simulink model "IDMF_datagenerator"  (R2022a)
settings: Solver=VariableStepAuto  StartTime=0.0  StopTime=30  FixedStep=0.05  RelTol=1e-3
PostLoadFcn:
  | %Add subfolders to path
  | addpath('virtualworld');
InitFcn:
  | startScript;
values from neighbouring files (symbols this model uses):
  angularVelocity = [0 0 -0.01]    [startScript.m]
  angularVelocityforLanding = [0 0 0]    [startScript.m]
  dronestartlocation = [-1.5 0 4]    [startScript.m]
  Dstar = -0.5    [startScript.m]
  finalHoverHeight = 2.5    [startScript.m]
  helipadLocation = [14 0.6 5]    [startScript.m]
  linearVelocity = [5 0.05 1]    [startScript.m]
  linearVelocityforHover = [0.65 0.05 0.3]    [startScript.m]
  windAVelocity = [0 0.1 0.1]    [startScript.m]
  windLVelocity = [0.1 0 0.3]    [startScript.m]
undefined symbols (not defined in the file or in its folder): fspecial, gcbh, Kanade, Lucas, Rec, SDTV, vrmfunc
libraries: visiontextngfix x11, visionconversions x9, visionanalysis x8, vrlib x7, slpidlib x3, sharedtransform x2, simulink x1
(part 3 of 3)

== matlab function IDMF_datagenerator/ Optical Flow Algorithm for Obstacle Avoidance/Subsystem/MATLAB Function4 ==
  data: points input; vel_Lines output single size=[5000 4]; vel_points output single size=[5000 2]
function [vel_Lines, vel_points]=OpticalFlowLines(points)
%persistent vel_Lines;
rop=round(points*100)/100;
orderedpoints = sortrows(rop);
orderedpoints1 = sortrows(rop,2);
X = [];
Y = [];
shiftX = [];
shiftY=[];
length(orderedpoints)
%(orderedpoints(i,1)==orderedpoints(i+1,1)|| orderedpoints(i,1)==orderedpoints(i+1,1)+1 || orderedpoints(i,1)==orderedpoints(i+1,1)-1 ...
                %|| orderedpoints(i,1)==orderedpoints(i+1,1)+2 || orderedpoints(i,1)==orderedpoints(i+1,1)-2) &&
%|| orderedpoints(i,1)==orderedpoints(i+1,1)+1 || orderedpoints(i,1)==orderedpoints(i+1,1)-1)
if length(orderedpoints)>2
for i = 1:2:length(orderedpoints)-1
    if i ==1 && orderedpoints(i,1)==orderedpoints(i+1,1)
        X = [X ;orderedpoints(i,1)];
        Y = [Y ;orderedpoints(i,2)];
        shiftX = [shiftX ;orderedpoints(i+1,1)];
        shiftY = [shiftY ;orderedpoints(i+1,2)];
    else
        if i ~=1 && (abs(orderedpoints(i,1)-orderedpoints(i+1,1))<3)
        X = [X ;orderedpoints(i,1)];
        Y = [Y ;orderedpoints(i,2)];
        shiftX = [shiftX ;orderedpoints(i+1,1)];
        shiftY = [shiftY ;orderedpoints(i+1,2)];
        
        elseif i~=1 &&  (abs(orderedpoints(i,1)-orderedpoints(i-1,1))<2)
        X = [X ;orderedpoints(i,1)];
        Y = [Y ;orderedpoints(i,2)];
        shiftX = [shiftX ;orderedpoints(i-1,1)];
        shiftY = [shiftY ;orderedpoints(i-1,2)];
    end
    end
end
for i = 1:2:length(orderedpoints1)-1
    if i ==1 && orderedpoints1(i,2)==orderedpoints1(i+1,2)
        X = [X ;orderedpoints1(i,1)];
        Y = [Y ;orderedpoints1(i,2)];
        shiftX = [shiftX ;orderedpoints1(i+1,1)];
        shiftY = [shiftY ;orderedpoints1(i+1,2)];
    else
        if i ~=1 && (abs(orderedpoints1(i,2)-orderedpoints1(i+1,2))<3)
        X = [X ;orderedpoints1(i,1)];
        Y = [Y ;orderedpoints1(i,2)];
        shiftX = [shiftX ;orderedpoints1(i+1,1)];
        shiftY = [shiftY ;orderedpoints1(i+1,2)];
        
        elseif i~=1 &&  (abs(orderedpoints1(i,2)-orderedpoints1(i-1,2))<2)
        X = [X ;orderedpoints1(i,1)];
        Y = [Y ;orderedpoints1(i,2)];
        shiftX = [shiftX ;orderedpoints1(i-1,1)];
        shiftY = [shiftY ;orderedpoints1(i-1,2)];
    end
    end
end
% for i = 1:length(orderedpoints)-1
%     for j=i+1:length(orderedpoints)
%         X = [X ;orderedpoints(i,1)];
%         Y = [Y ;orderedpoints(i,2)];
%         shiftX = [shiftX ;orderedpoints(j,1)];
%         shiftY = [shiftY ;orderedpoints(j,2)];
%     end
% end

    vel_points = [X(:), Y(:); shiftX(:),  shiftY(:) ];
    x= single([X(:), Y(:), shiftX(:),  shiftY(:)]);

else
    vel_points = [points; points];
    x= single([points, points]);
end
vel_Lines=x;
% vel_Lines=padarray(x,50-length(x),0,'post');

== matlab function IDMF_datagenerator/ Optical Flow Algorithm for Obstacle Avoidance/Subsystem/sumele ==
  data: u input; y1 output; n1 output; y2 output; n2 output
function [y1,n1,y2,n2] = fcn(u)
u1=rmoutliers(u);
u2=rmoutliers(u,'percentiles',[30 70]);
n1=length(u1);
n2=length(u2);
% if n1==1
%     y1=0.00;
% else
y1 = double(sum(u1));
% end
y2 = double(sum(u2));
if n2==1
    y2=0.00;
else
y2 = double(sum(u2))/n2;
end

== matlab function IDMF_datagenerator/ Optical Flow Algorithm for Obstacle Avoidance/Subsystem/length1 ==
  data: lines input; l1 output size=5000; l2 output size=5000; N output; reset input; oldlines output size=[5000 4]
function [l1,l2,N,oldlines] = fcn(lines, reset)
l1=single([]);
l2=single([]);
persistent x;
% size(x)
if isempty(x)
    x=lines;
end
if reset>0
    oldlines=x;
else
    oldlines=lines;
end
N = 0;
% size(lines)
if isempty(nonzeros(oldlines))
    oldlines=lines;
end

a1=size(lines);
a1=a1(1,1);
a2=size(oldlines);
a2=a2(1,1);
lines = sortrows(lines);
oldlines=sortrows(oldlines);
% a1=length(lines);
% a2=length(oldlines);
if a1<=a2
for i = 1: a1
    for j = 1:a2
        if abs(lines(i,1) + lines(i,3) - oldlines(j,3) -oldlines(j,1))<=5 && N~=i
           if norm(lines(i,1:2)-lines(i,3:4))~=0 && norm(oldlines(j,1:2)-oldlines(j,3:4))~=0
            l1 = [l1 ;norm(lines(i,1:2)-lines(i,3:4))];
            l2 = [l2; norm(oldlines(j,1:2)-oldlines(j,3:4))];
            N = N+1;
           end
        end
    end
end
else
for i = 1: a2
    for j = 1:a1
        if abs(oldlines(i,1) + oldlines(i,3) - lines(j,3) -lines(j,1))<=5  && N~=i
           if norm(lines(j,1:2)-lines(j,3:4))~=0 && norm(oldlines(i,1:2)-oldlines(i,3:4))~=0
            l1 = [l1 ;norm(lines(j,1:2)-lines(j,3:4))];
            l2 = [l2; norm(oldlines(i,1:2)-oldlines(i,3:4))];
            N = N+1;
           end
        end
    end
end
end
x=lines;

== matlab function IDMF_datagenerator/ Optical Flow Algorithm for Obstacle Avoidance/Subsystem/length2 ==
  data: lines input; oldlines input; l1 output size=5000; l2 output size=5000; N output
function [l1,l2,N] = fcn(lines,oldlines)
l1=single([]);
l2=single([]);
% persistent x;
% % size(x)
% if isempty(x)
%     x=lines;
% end
% if reset>0
%     oldlines=x;
% else
%     oldlines=lines;
% end
N = 0;
% % size(lines)
% if isempty(nonzeros(oldlines))
%     oldlines=lines;
% end

a1=size(lines);
a1=a1(1,1);
a2=size(oldlines);
a2=a2(1,1);
lines = sortrows(lines);
oldlines=sortrows(oldlines);
% a1=length(lines);
% a2=length(oldlines);
if a1<=a2
for i = 1: a1
    for j = i:a2
        if abs(lines(i,1) + lines(i,3) - oldlines(j,3) -oldlines(j,1))<=7 && N~=i
           if norm(lines(i,1:2)-lines(i,3:4))~=0 && norm(oldlines(j,1:2)-oldlines(j,3:4))~=0 ...
%                    && norm(lines(i,1:2)-lines(i,3:4))>=norm(oldlines(j,1:2)-oldlines(j,3:4))
            l1 = [l1 ;norm(lines(i,1:2)-lines(i,3:4))];
            l2 = [l2; norm(oldlines(j,1:2)-oldlines(j,3:4))];
            N = N+1;
           end
        end
    end
end
else
for i = 1: a2
    for j = i:a1
        if abs(oldlines(i,1) + oldlines(i,3) - lines(j,3) -lines(j,1))<=7  && N~=i
           if norm(lines(j,1:2)-lines(j,3:4))~=0 && norm(oldlines(i,1:2)-oldlines(i,3:4))~=0 ...
%                    && norm(lines(j,1:2)-lines(j,3:4))>=norm(oldlines(i,1:2)-oldlines(i,3:4))
            l1 = [l1 ;norm(lines(j,1:2)-lines(j,3:4))];
            l2 = [l2; norm(oldlines(i,1:2)-oldlines(i,3:4))];
            N = N+1;
           end
        end
    end
end
end
x=lines;

== matlab function IDMF_datagenerator/ Optical Flow Algorithm for Obstacle Avoidance/Subsystem/MATLAB Function6 ==
  data: points input; old_Lines output single size=[5000 4]; vel_points output single size=[5000 2]
function [old_Lines, vel_points]=OpticalFlowLines(points)
%persistent vel_Lines;
rop=round(points*100)/100;
orderedpoints = sortrows(rop);
orderedpoints1 = sortrows(rop,2);
X = [];
Y = [];
shiftX = [];
shiftY=[];
% length(orderedpoints)
%(orderedpoints(i,1)==orderedpoints(i+1,1)|| orderedpoints(i,1)==orderedpoints(i+1,1)+1 || orderedpoints(i,1)==orderedpoints(i+1,1)-1 ...
                %|| orderedpoints(i,1)==orderedpoints(i+1,1)+2 || orderedpoints(i,1)==orderedpoints(i+1,1)-2) &&
%|| orderedpoints(i,1)==orderedpoints(i+1,1)+1 || orderedpoints(i,1)==orderedpoints(i+1,1)-1)
if length(orderedpoints)>2
for i = 1:2:length(orderedpoints)-1
    if i ==1 && orderedpoints(i,1)==orderedpoints(i+1,1)
        X = [X ;orderedpoints(i,1)];
        Y = [Y ;orderedpoints(i,2)];
        shiftX = [shiftX ;orderedpoints(i+1,1)];
        shiftY = [shiftY ;orderedpoints(i+1,2)];
    else
        if i ~=1 && (abs(orderedpoints(i,1)-orderedpoints(i+1,1))<3)
        X = [X ;orderedpoints(i,1)];
        Y = [Y ;orderedpoints(i,2)];
        shiftX = [shiftX ;orderedpoints(i+1,1)];
        shiftY = [shiftY ;orderedpoints(i+1,2)];
        
        elseif i~=1 &&  (abs(orderedpoints(i,1)-orderedpoints(i-1,1))<2)
        X = [X ;orderedpoints(i,1)];
        Y = [Y ;orderedpoints(i,2)];
        shiftX = [shiftX ;orderedpoints(i-1,1)];
        shiftY = [shiftY ;orderedpoints(i-1,2)];
    end
    end
end
for i = 1:2:length(orderedpoints1)-1
    if i ==1 && orderedpoints1(i,2)==orderedpoints1(i+1,2)
        X = [X ;orderedpoints1(i,1)];
        Y = [Y ;orderedpoints1(i,2)];
        shiftX = [shiftX ;orderedpoints1(i+1,1)];
        shiftY = [shiftY ;orderedpoints1(i+1,2)];
    else
        if i ~=1 && (abs(orderedpoints1(i,2)-orderedpoints1(i+1,2))<3)
        X = [X ;orderedpoints1(i,1)];
        Y = [Y ;orderedpoints1(i,2)];
        shiftX = [shiftX ;orderedpoints1(i+1,1)];
        shiftY = [shiftY ;orderedpoints1(i+1,2)];
        
        elseif i~=1 &&  (abs(orderedpoints1(i,2)-orderedpoints1(i-1,2))<2)
        X = [X ;orderedpoints1(i,1)];
        Y = [Y ;orderedpoints1(i,2)];
        shiftX = [shiftX ;orderedpoints1(i-1,1)];
        shiftY = [shiftY ;orderedpoints1(i-1,2)];
    end
    end
end
% for i = 1:length(orderedpoints)-1
%     for j=i+1:length(orderedpoints)
%         X = [X ;orderedpoints(i,1)];
%         Y = [Y ;orderedpoints(i,2)];
%         shiftX = [shiftX ;orderedpoints(j,1)];
%         shiftY = [shiftY ;orderedpoints(j,2)];
%     end
% end

    vel_points = [X(:), Y(:); shiftX(:),  shiftY(:) ];
    x= single([X(:), Y(:), shiftX(:),  shiftY(:)]);

else
    vel_points = [points; points];
    x= single([points, points]);
end
old_Lines=x;
% vel_Lines=padarray(x,50-length(x),0,'post');

== matlab function IDMF_datagenerator/ Optical Flow Algorithm for Obstacle Avoidance/Subsystem/Combo ==
  data: newpoints input; New_Lines output size=[2000,4]; oldpoints input; Old_Lines output size=[2000,4]
function [New_Lines, Old_Lines] = fcn(newpoints,oldpoints)


rop=round(newpoints*100)/100;
rop1=round(oldpoints*100)/100;

X = [];
Y = [];
shiftX = [];
shiftY=[];
X1 = [];
Y1 = [];
shiftX1 = [];
shiftY1=[];
%(orderedpoints(i,1)==orderedpoints(i+1,1)|| orderedpoints(i,1)==orderedpoints(i+1,1)+1 || orderedpoints(i,1)==orderedpoints(i+1,1)-1 ...
                %|| orderedpoints(i,1)==orderedpoints(i+1,1)+2 || orderedpoints(i,1)==orderedpoints(i+1,1)-2) &&
%|| orderedpoints(i,1)==orderedpoints(i+1,1)+1 || orderedpoints(i,1)==orderedpoints(i+1,1)-1)


% if length(orderedpoints)>2
% for i = 1:2:length(orderedpoints)-1
%     if i ==1 && orderedpoints(i,1)==orderedpoints(i+1,1)
%         X = [X ;orderedpoints(i,1)];
%         Y = [Y ;orderedpoints(i,2)];
%         shiftX = [shiftX ;orderedpoints(i+1,1)];
%         shiftY = [shiftY ;orderedpoints(i+1,2)];
% 
%         X1 = [X1 ;orderedpoints1(i,1)];
%         Y1 = [Y1 ;orderedpoints1(i,2)];
%         shiftX1 = [shiftX1 ;orderedpoints1(i+1,1)];
%         shiftY1 = [shiftY1 ;orderedpoints1(i+1,2)];
%     else
%         if i ~=1 && (abs(orderedpoints(i,1)-orderedpoints(i+1,1))<3)
%         X = [X ;orderedpoints(i,1)];
%         Y = [Y ;orderedpoints(i,2)];
%         shiftX = [shiftX ;orderedpoints(i+1,1)];
%         shiftY = [shiftY ;orderedpoints(i+1,2)];
% 
%         X1 = [X1 ;orderedpoints1(i,1)];
%         Y1 = [Y1 ;orderedpoints1(i,2)];
%         shiftX1 = [shiftX1 ;orderedpoints1(i+1,1)];
%         shiftY1 = [shiftY1 ;orderedpoints1(i+1,2)];
%         
%         elseif i~=1 &&  (abs(orderedpoints(i,1)-orderedpoints(i-1,1))<2)
%         X = [X ;orderedpoints(i,1)];
%         Y = [Y ;orderedpoints(i,2)];
%         shiftX = [shiftX ;orderedpoints(i-1,1)];
%         shiftY = [shiftY ;orderedpoints(i-1,2)];
% 
%         X1 = [X1 ;orderedpoints1(i,1)];
%         Y1 = [Y1 ;orderedpoints1(i,2)];
%         shiftX1 = [shiftX1 ;orderedpoints1(i-1,1)];
%         shiftY1 = [shiftY1 ;orderedpoints1(i-1,2)];
%     end
%     end
% end
% for i = 1:2:length(orderedpoints2)-1
%     if i ==1 && orderedpoints2(i,2)==orderedpoints2(i+1,2)
%         X = [X ;orderedpoints2(i,1)];
%         Y = [Y ;orderedpoints2(i,2)];
%         shiftX = [shiftX ;orderedpoints2(i+1,1)];
%         shiftY = [shiftY ;orderedpoints2(i+1,2)];
% 
%         X1 = [X1 ;orderedpoints3(i,1)];
%         Y1 = [Y1 ;orderedpoints3(i,2)];
%         shiftX1 = [shiftX1 ;orderedpoints3(i+1,1)];
%         shiftY1 = [shiftY1 ;orderedpoints3(i+1,2)];
% 
%     else
%         if i ~=1 && (abs(orderedpoints2(i,2)-orderedpoints2(i+1,2))<3)
%         X = [X ;orderedpoints2(i,1)];
%         Y = [Y ;orderedpoints2(i,2)];
%         shiftX = [shiftX ;orderedpoints2(i+1,1)];
%         shiftY = [shiftY ;orderedpoints2(i+1,2)];
% 
%         X1 = [X1 ;orderedpoints3(i,1)];
%         Y1 = [Y1 ;orderedpoints3(i,2)];
%         shiftX1 = [shiftX1 ;orderedpoints3(i+1,1)];
%         shiftY1 = [shiftY1 ;orderedpoints3(i+1,2)];
%         
%         elseif i~=1 &&  (abs(orderedpoints2(i,2)-orderedpoints2(i-1,2))<2)
%         X = [X ;orderedpoints2(i,1)];
%         Y = [Y ;orderedpoints2(i,2)];
%         shiftX = [shiftX ;orderedpoints2(i-1,1)];
%         shiftY = [shiftY ;orderedpoints2(i-1,2)];
% 
%         X1 = [X1 ;orderedpoints3(i,1)];
%         Y1 = [Y1 ;orderedpoints3(i,2)];
%         shiftX1 = [shiftX1 ;orderedpoints3(i-1,1)];
%         shiftY1 = [shiftY1 ;orderedpoints3(i-1,2)];
%     end
%     end
% end
% % for i = 1:length(orderedpoints)-1
% %     for j=i+1:length(orderedpoints)
% %         X = [X ;orderedpoints(i,1)];
% %         Y = [Y ;orderedpoints(i,2)];
% %         shiftX = [shiftX ;orderedpoints(j,1)];
% %         shiftY = [shiftY ;orderedpoints(j,2)];
% %     end
% % end
% 
%     vel_points = [X(:), Y(:); shiftX(:),  shiftY(:) ];
%     x= single([X(:), Y(:), shiftX(:),  shiftY(:)]);
% 
%     vel_points1 = [X1(:), Y1(:); shiftX1(:),  shiftY1(:) ];
%     x1= single([X1(:), Y1(:), shiftX1(:),  shiftY1(:)]);
% else
%     vel_points = [newpoints; newpoints];
%     x= single([newpoints, newpoints]);
% 
%     vel_points1 = [oldpoints; oldpoints];
%     x1= single([oldpoints, oldpoints]);
% end

for i = 1:length(newpoints)
    for j= i+1:length(newpoints)
        if abs(newpoints(i,1)-newpoints(j,1))<1
            X = [X ;newpoints(i,1)];
            Y = [Y ;newpoints(i,2)];
            shiftX = [shiftX ;newpoints(j,1)];
            shiftY = [shiftY ;newpoints(j,2)];

            X1 = [X1 ;oldpoints(i,1)];
            Y1 = [Y1 ;oldpoints(i,2)];
            shiftX1 = [shiftX1 ;oldpoints(j,1)];
            shiftY1 = [shiftY1 ;oldpoints(j,2)];
        end
    end
end

for i = 1:length(newpoints)
    for j= i+1:length(newpoints)
        if abs(newpoints(i,2)-newpoints(j,2))<2
            X = [X ;newpoints(i,1)];
            Y = [Y ;newpoints(i,2)];
            shiftX = [shiftX ;newpoints(j,1)];
            shiftY = [shiftY ;newpoints(j,2)];

            X1 = [X1 ;oldpoints(i,1)];
            Y1 = [Y1 ;oldpoints(i,2)];
            shiftX1 = [shiftX1 ;oldpoints(j,1)];
            shiftY1 = [shiftY1 ;oldpoints(j,2)];
        end
    end
end
New_Lines=single([X(:), Y(:), shiftX(:),  shiftY(:)]);
Old_Lines=single([X1(:), Y1(:), shiftX1(:),  shiftY1(:)]);
